simulink model "ThreePhase"  (R2023b)
settings: Solver=ode45  StartTime=0.0  StopTime=0.06  RelTol=1e-3
libraries: spsCurrentMeasurementLib x4, spsThyristorLib x3, spsACVoltageSourceLib x3, spsSeriesRLCBranchLib x1, spsVoltageMeasurementLib x1, sps_lib x1
settings Model: Creator=Ayman Tarek  LastModifiedBy=Ayman Tarek

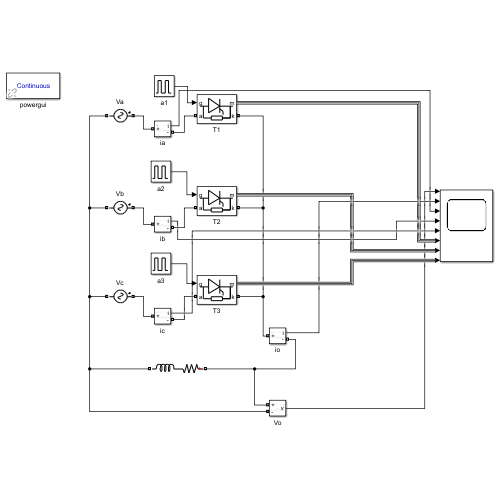
[thumbnail: Simulink's stored preview of the top-level diagram]
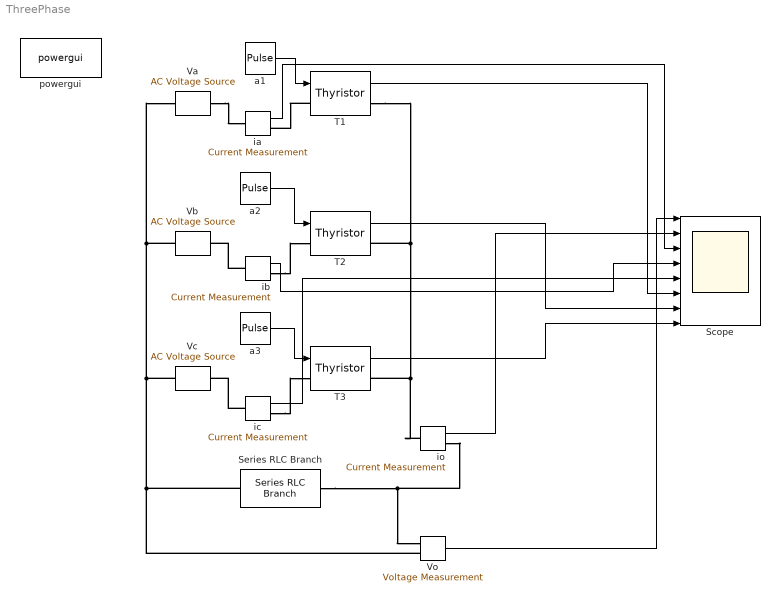
== system ThreePhase ==
  Scope : Scope  NumInputPorts=8
  Series RLC Branch : spsSeriesRLCBranchLib/Series RLC Branch  LConnTagsString=__new0  RConnTagsString=__new0  BranchType=RL  Resistance=5  Inductance=0.02  SetiL0=off  InitialCurrent=0  Capacitance=0  Setx0=off  InitialVoltage=0  Measurements=None
  T1 : spsThyristorLib/Thyristor  Ron=0  Lon=0  Vf=0  IC=0  Rs=500  Cs=250e-9  Measurements=on
  T2 : spsThyristorLib/Thyristor  Ron=0  Lon=0  Vf=0  IC=0  Rs=500  Cs=250e-9  Measurements=on
  T3 : spsThyristorLib/Thyristor  Ron=0  Lon=0  Vf=0  IC=0  Rs=500  Cs=250e-9  Measurements=on
  Va : spsACVoltageSourceLib/AC Voltage Source  Amplitude=50  Phase=0  Frequency=50  SampleTime=0  Measurements=None  BusType=swing  Pref=10e3  Qref=0  Qmin=-inf  Qmax=+inf
  Vb : spsACVoltageSourceLib/AC Voltage Source  Amplitude=50  Phase=-120  Frequency=50  SampleTime=0  Measurements=None  BusType=swing  Pref=10e3  Qref=0  Qmin=-inf  Qmax=+inf
  Vc : spsACVoltageSourceLib/AC Voltage Source  Amplitude=50  Phase=120  Frequency=50  SampleTime=0  Measurements=None  BusType=swing  Pref=10e3  Qref=0  Qmin=-inf  Qmax=+inf
  Vo : spsVoltageMeasurementLib/Voltage Measurement  PhasorSimulation=off  OutputType=Complex  PSBequivalent=0
  a1 : DiscretePulseGenerator  PulseType=Time based  Period=0.02  PulseWidth=10  PhaseDelay=((30+60)*0.02)/360
  a2 : DiscretePulseGenerator  PulseType=Time based  Period=0.02  PulseWidth=10  PhaseDelay=((150+60)*0.02)/360
  a3 : DiscretePulseGenerator  PulseType=Time based  Period=0.02  PulseWidth=10  PhaseDelay=((270+60)*0.02)/360
  ia : spsCurrentMeasurementLib/Current Measurement  PhasorSimulation=off  OutputType=Complex  PSBequivalent=0
  ib : spsCurrentMeasurementLib/Current Measurement  PhasorSimulation=off  OutputType=Complex  PSBequivalent=0
  ic : spsCurrentMeasurementLib/Current Measurement  PhasorSimulation=off  OutputType=Complex  PSBequivalent=0
  io : spsCurrentMeasurementLib/Current Measurement  PhasorSimulation=off  OutputType=Complex  PSBequivalent=0
  powergui : sps_lib/powergui  Priority=1  SimulationMode=Continuous  SampleTime=50e-6  frequency=60  Iterations=50  frequencyindice=50  Pbase=100e6  ErrMax=1e-4  UnitsV=kV  UnitsW=MW  buscounter=0  FunctionMessages=off  echomessages=off  EnableUseOfTLC=off  CurrentSourceSwitches=off  DisableSnubberDevices=off  DisableRonSwitches=off  DisableVfSwitches=off  DisplayEquations=off  AutomaticDiscreteSolvers=off  SolverType=Tustin/Backward Euler (TBE)  Interpol=off  ExternalGateDelay=off  methode=off  Ts=100  x0status=blocks  SPID=on  SwTol=0  HookPort=off  NonlinearTolerance=1e-4  nMaxIteration=100  ContinueOnMaxIteration=off  RestoreLinks=warning  ResistiveCurrentMeasurement=off  Frange=[0:2:500]  Ylog=off  Xlog=on  ShowGrid=off  save=off  variable=ZData  structure=0  ZoomFFT=off  StartTime=0.0  cycles=1  DisplayStyle=1  fundamental=60  FreqAxis=off  MaxFrequency=1000  frequencyindicesteady=1  RmsSteady=1  display=off
  wires:
  a1/1 -> T1/1
  a2/1 -> T2/1
  a3/1 -> T3/1
  Vo/1 -> Scope/1
  io/1 -> Scope/2
  ia/1 -> Scope/3
  ib/1 -> Scope/4
  ic/1 -> Scope/5
  T1/1 -> Scope/6
  T2/1 -> Scope/7
  T3/1 -> Scope/8
  connections:
  Vb/LConn1 -- Va/LConn1 -- Vo/LConn2 -- Series RLC Branch/RConn1 -- Vc/LConn1
  T1/RConn1 -- io/LConn1 -- T3/RConn1 -- T2/RConn1
  Va/RConn1 -- ia/LConn1
  T1/LConn1 -- ia/RConn1
  ib/LConn1 -- Vb/RConn1
  ib/RConn1 -- T2/LConn1
  ic/LConn1 -- Vc/RConn1
  ic/RConn1 -- T3/LConn1
  Series RLC Branch/LConn1 -- io/RConn1 -- Vo/LConn1
